simulink library "AP_Conector"  (R2025b)
settings: Solver=VariableStepAuto  StartTime=0.0  StopTime=10.0  RelTol=1e-3
settings Model: Creator=Peter  LastModifiedBy=luke.miller
settings SolverCC: AlgebraicLoopSolver=TrustRegion
settings DebuggingCC: UnconnectedInputMsg=warning  UnconnectedOutputMsg=warning  UnconnectedLineMsg=warning
settings ModelReferenceCC: EnableRefExpFcnMdlSchedulingChecks=on
settings RTWCC: GPUComputeCapability=3.5

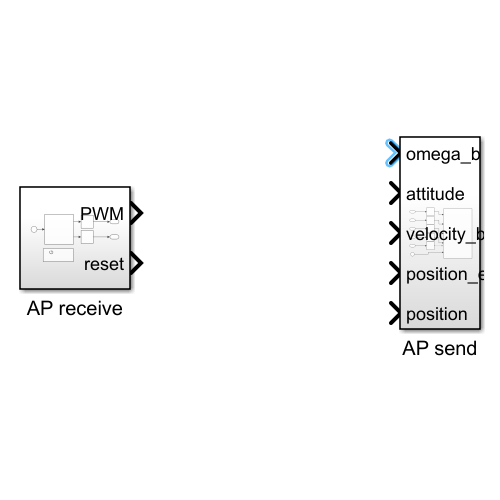
[thumbnail: Simulink's stored preview of the top-level diagram]
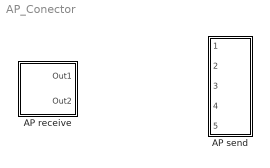
== system AP_Conector ==
  AP receive : Subsystem
  AP send : Subsystem

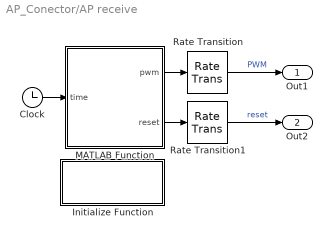
== system AP_Conector/AP receive ==
  Clock : Clock
  Initialize Function : Subsystem  TreatAsAtomicUnit=on
  MATLAB Function : MATLAB Function  TreatAsAtomicUnit=on  SystemSampleTime=1/400
  Rate Transition : RateTransition
  Rate Transition1 : RateTransition
  Out1 : Outport
  Out2 : Outport  Port=2
  wires:
  Rate Transition/1 -> Out1/1  "PWM"
  MATLAB Function/1(pwm) -> Rate Transition/1
  Clock/1 -> MATLAB Function/1(time)
  MATLAB Function/2(reset) -> Rate Transition1/1
  Rate Transition1/1 -> Out2/1  "reset"

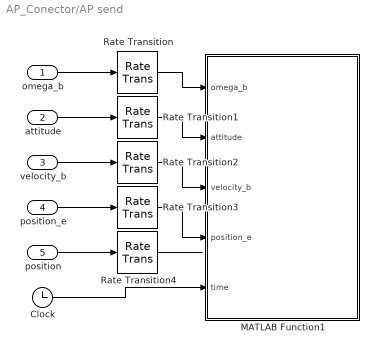
== system AP_Conector/AP send ==
  omega_b : Inport
  attitude : Inport  Port=2
  velocity_b : Inport  Port=3
  position_e : Inport  Port=4
  position : Inport  Port=5
  Clock : Clock
  MATLAB Function1 : MATLAB Function  TreatAsAtomicUnit=on  SystemSampleTime=1/400
  Rate Transition{,1..4} (5 alike) : RateTransition
  wires:
  attitude/1 -> Rate Transition1/1
  omega_b/1 -> Rate Transition/1
  Rate Transition/1 -> MATLAB Function1/1(omega_b)
  Clock/1 -> MATLAB Function1/5(time)
  Rate Transition3/1 -> MATLAB Function1/4(position_e)
  Rate Transition2/1 -> MATLAB Function1/3(velocity_b)
  Rate Transition1/1 -> MATLAB Function1/2(attitude)
  velocity_b/1 -> Rate Transition2/1
  Rate Transition4/1 -> ?
  position_e/1 -> Rate Transition3/1
  position/1 -> Rate Transition4/1

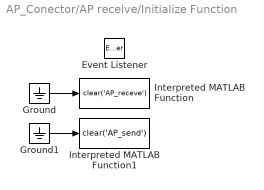
== system AP_Conector/AP receive/Initialize Function ==
  Event Listener : EventListener  DisableCoverage=on  EventName=reset
  Ground : Ground
  Ground1 : Ground
  Interpreted MATLAB Function : MATLABFcn  MATLABFcn=clear('AP_receve')  OutputDimensions=0
  Interpreted MATLAB Function1 : MATLABFcn  MATLABFcn=clear('AP_send')  OutputDimensions=0
  wires:
  Ground1/1 -> Interpreted MATLAB Function1/1
  Ground/1 -> Interpreted MATLAB Function/1

== matlab function AP_Conector/AP receive/MATLAB Function ==
  data: pwm output; time input; reset output
function [pwm, reset] = fcn(time)
%#codegen

pwm = zeros(1,16);
reset = false;

coder.extrinsic('AP_receve');

[pwm_temp, reset_temp] = AP_receve(time);

pwm = pwm_temp;
reset = reset_temp;

end

== matlab function AP_Conector/AP send/MATLAB Function1 ==
  data: omega_b input; attitude input; velocity_b input; position_e input; time input
function sendToAP(omega_b, attitude, velocity_b, position_e, time)

coder.extrinsic('AP_send');

AP_send(omega_b, attitude, velocity_b, position_e, time);

end
